simulink model "modelControl"  (R2024b)
settings: Solver=FixedStepAuto  StartTime=0  StopTime=stopTime  FixedStep=dt  RelTol=1e-3
values from neighbouring files (symbols this model uses):
  A = -1/(R*c)    [RealTimeSim.m]    (also in fridge_fixed_step.m)
  B = [1/(R),G]    [RealTimeSim.m]    (also in fridge_fixed_step.m = [G,1/R])
  C = 1/c    [RealTimeSim.m]    (also in fridge_fixed_step.m)
  D = [0,0]    [RealTimeSim.m]    (also in fridge_fixed_step.m)
  th = -22    [RealTimeSim.m]
  th2 = -20    [RealTimeSim.m]
undefined symbols (not defined in the file or in its folder): hysteresis, x0
settings Model: Creator=mikol  LastModifiedBy=mikol

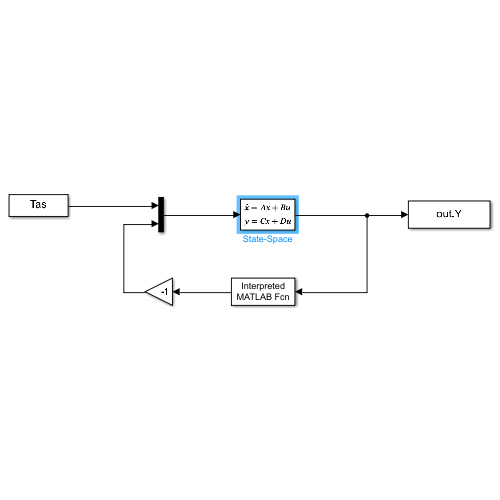
[thumbnail: Simulink's stored preview of the top-level diagram]
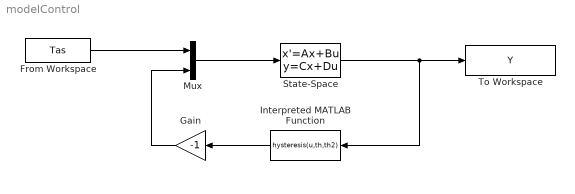
== system modelControl ==
  From Workspace : FromWorkspace  VariableName=Tas
  Gain : Gain  Gain=-1
  Interpreted MATLAB Function : MATLABFcn  MATLABFcn=hysteresis(u,th,th2)  OutputDimensions=1
  Mux : Mux  Inputs=2
  State-Space : StateSpace  A=A  B=B  C=C  D=D  InitialCondition=x0
  To Workspace : ToWorkspace  VariableName=Y  SaveFormat=Timeseries  SampleTime=-1
  wires:
  Mux/1 -> State-Space/1
  From Workspace/1 -> Mux/1
  State-Space/1 -> To Workspace/1, Interpreted MATLAB Function/1
  Interpreted MATLAB Function/1 -> Gain/1
  Gain/1 -> Mux/2
